simulink model "simVSG"  (R2023a)
settings: Solver=VariableStepAuto  StartTime=0.0  StopTime=Tend  MaxStep=Ts/3  RelTol=1e-3
values from neighbouring files (symbols this model uses):
  Cf = 1.3157e-4    (= 0.00013157)    [VSG.m]
  Dp0 = 3    [VSG.m]
  Fg = 50    [VSG.m]
  Fsw = 2.5e3    (= 2500)    [VSG.m]
  J0 = 3.0/Jn    (= 1.23370055014)    [VSG.m]
  Kd = 150    [VSG.m]
  Kii = Rf*alpha_i / Zn    (= 0.654498469498)    [VSG.m]
  Kj = 30    [VSG.m]
  Kpi = Lf*alpha_i / Zn    (= 0.208332452222)    [VSG.m]
  Kpv = alpha_v*sqrt(alpha_v^2+alpha_i^2)/alpha_i *Zn    [VSG.m]
  Lf = 5.7773e-4    (= 0.00057773)    [VSG.m]
  Pn = 120    [VSG.m]
  Rf = 1.815e-3    (= 0.001815)    [VSG.m]
  Ts = 5e-05    [VSG.m]
  Udc = 800    [VSG.m]
  Ug = 220    [VSG.m]
  Z1 = .09 + 1j*.12    [VSG.m]
  Z3 = .1 + 1j*1.5    [VSG.m]
  Zn = 3*Ug^2 / Pn/1e3    (= 1.21)    [VSG.m]
undefined symbols (not defined in the file or in its folder): DiscIntNeverNeededParam, Vnom_prim
libraries: spsSecondOrderFilterLib x8, simulink x8, spsFirstOrderFilterLib x6, spsThreePhaseSeriesRLCBranchLib x4, spsThreePhaseSeriesRLCLoadLib x3, slpidlib x3, spsThreePhaseVIMeasurementLib x3, spsGroundLib x2, spsPowerPLLDrivenPositiveSequenceLib x2, spsabctodq0Lib x2, spsFundamentalPLLDrivenLib x2, spsPLL3phLib x2
(part 1 of 2)
settings Model: Creator=si  LastModifiedBy=si

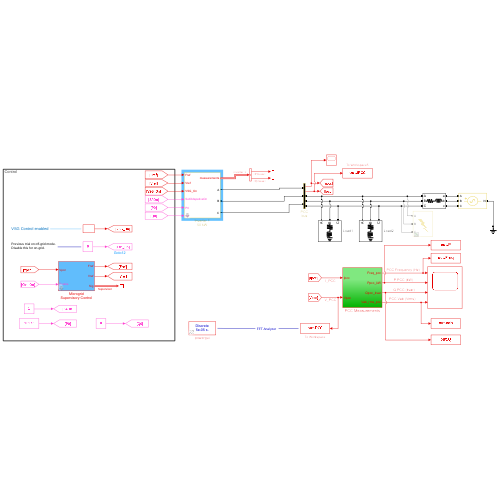
[thumbnail: Simulink's stored preview of the top-level diagram]
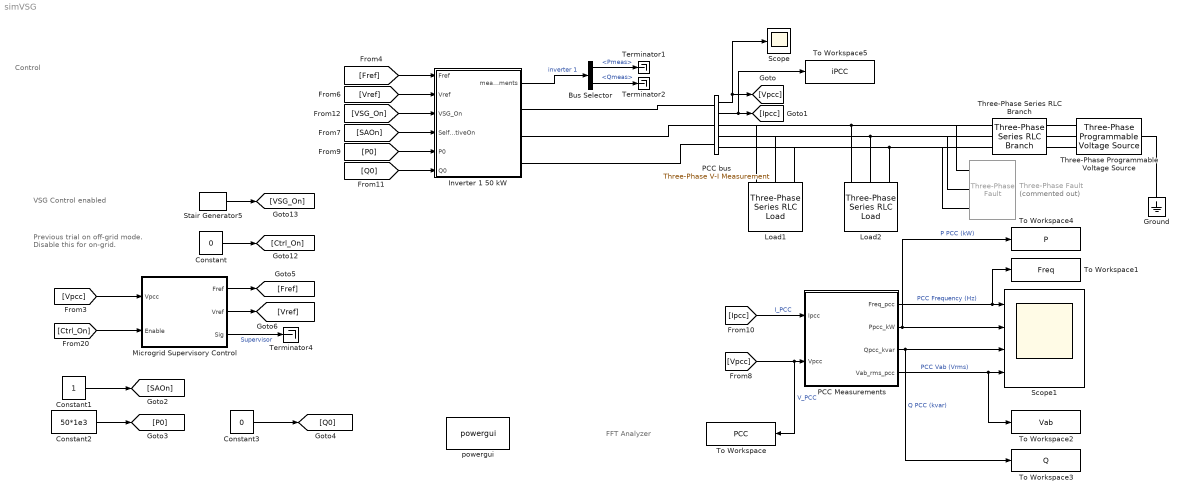
== system simVSG ==
  note: Previous trial on off-grid mode. Disable this for on-grid.
  note: VSG Control enabled
  note: Control
  note: FFT Analyzer
  Bus Selector : BusSelector  OutputSignals=Control.Pmeas,Control.Qmeas
  Constant : Constant  Value=0
  Constant1 : Constant
  Constant2 : Constant  Value=50*1e3
  Constant3 : Constant  Value=0
  Ground : spsGroundLib/Ground  LConnTagsString=a
  Inverter 1 50 kW : Subsystem  mask(Grid-Forming Inverter with droop control){Pnom=Pn*1e3, Fnom=Fg, Vnom=Ug*sqrt(3), Vnom_dc=Udc, Frequency_Droop=25, Voltage_Droop=10, Kp_Vreg=Kpv, Ki_Vreg=0, Kp_Ireg=Kpi, Ki_Ireg=Kii, RLff=[ Rf/Zn, Lf/Zn*2*pi], Fsw=Fsw, CarrierPhase=90, fn_Filter=400, Ts=Ts, ZL=Z1, J0=J0, Dp0=Dp0, Kj=Kj, Kd=Kd, Lv=imag(Z1) / (2*pi*Fg), Rv=real(Z1)}
      mask prompts: Pnom "Power (VA)"; Fnom "Frequency (Hz)"; Vnom "Primary line voltage (Vrms)"; Vnom_dc "DC link voltage (V)"; Frequency_Droop "Frequency droop (%)"; Voltage_Droop "Voltage droop (%)"; Kp_Vreg "Proportional gain"; Ki_Vreg "Integral gain"; Kp_Ireg "Proportional gain"; Ki_Ireg "Integral gain"; RLff "Feedforward coefficients (pu)"; Fsw "Switching frequency (Hz)"; CarrierPhase "Carrier initial phase (degrees)"; fn_Filter "Measurement filters fn (Hz)"; Ts "Sample time (s)"; ZL "Line impedance"; J0 "Initial virtual inertia"; Dp0 "Initial damping factor"; Kj "Inertial changing rate Kj"; Kd "Damping factor changing rate Kd"; Lv "Virtual inductance"; Rv "Virtual resistance"
      mask init:
      | Rff=RLff(1);
      | Lff=RLff(2);
      mask DialogControl Container4 Prompt: Nominal Values:
      mask DialogControl Container8 Prompt: Droop Values
      mask DialogControl Container7 Prompt: Voltage Regulators
      mask DialogControl Container10 Prompt: Current Regulators
      mask DialogControl Ts1 Prompt: PWM Generator
      mask DialogControl Container9 Prompt: Line impedance
      mask DialogControl Container11 Prompt: VSG parameters
  Load1 : spsThreePhaseSeriesRLCLoadLib/Three-Phase Series RLC Load  LConnTagsString=A|B|C  Configuration=Y (grounded)  NominalVoltage=Ug*sqrt(3)  Vabc=[1e3 1e3 1e3]  Vabcp=[1e3 1e3 1e3]  NominalFrequency=Fg  UnbalancedPower=off  ActivePower=40e3  InductivePower=10e3  CapacitivePower=0  Pabc=[10e3 9e3 11e3]  QLabc=[100 90 110]  QCabc=[100 90 110]  Pabcp=[10e3 9e3 11e3]  QLabcp=[100 90 110]  QCabcp=[100 90 110]  Measurements=None  LoadType=constant Z
  Load2 : spsThreePhaseSeriesRLCLoadLib/Three-Phase Series RLC Load  LConnTagsString=A|B|C  Configuration=Y (grounded)  NominalVoltage=Ug*sqrt(3)  Vabc=[1e3 1e3 1e3]  Vabcp=[1e3 1e3 1e3]  NominalFrequency=Fg  UnbalancedPower=off  ActivePower=2e3  InductivePower=6e3  CapacitivePower=0  Pabc=[10e3 9e3 11e3]  QLabc=[100 90 110]  QCabc=[100 90 110]  Pabcp=[10e3 9e3 11e3]  QLabcp=[100 90 110]  QCabcp=[100 90 110]  Measurements=None  LoadType=constant Z
  Microgrid Supervisory Control : Subsystem  mask(Microgrid Supervisory Control){Fnom=Fg, Vnom=Ug*sqrt(3), Kp_Freg=0.03, Ki_Freg=2, Freg_Limits=[1.05, 0.95] * Fg, Kp_Vreg=0.1, Ki_Vreg=7, Vreg_Limits=[1.05, 0.95] * Ug*sqrt(3), fn_Filter=10, Ts=Ts}
      mask prompts: Fnom "Frequency (Hz)"; Vnom "Line voltage (Vrms)"; Kp_Freg "Proportional gain"; Ki_Freg "Integral gain"; Freg_Limits "Output limits (Hz): [Upper Lower]"; Kp_Vreg "Proportional gain"; Ki_Vreg "Integral gain"; Vreg_Limits "Output limits (Hz): [Upper Lower]"; fn_Filter "Measurement filter fn (Hz)"; Ts "Sample time (s)"
      mask DialogControl Container4 Prompt: Nominal Values:
      mask DialogControl Container7 Prompt: Frequency Regulator
      mask DialogControl Container10 Prompt: Voltage Regulator
  PCC bus : spsThreePhaseVIMeasurementLib/Three-Phase V-I Measurement  VoltageMeasurement=phase-to-ground  SetLabelV=off  LabelV=Vabc  Vpu=off  VpuLL=off  CurrentMeasurement=yes  SetLabelI=off  LabelI=Iabc  Ipu=off  Pbase=100e6  Vbase=500e3  OutputType=Complex  PhasorSimulation=off  PSBequivalent=0
  PCC Measurements : Subsystem
  Scope : Scope
  Scope1 : Scope  NumInputPorts=4
  Stair Generator5 : spsStairGeneratorLib/Stair Generator  t=[0, Ts]  e=[0, 1]  Ts=Ts
  Terminator1 : Terminator
  Terminator2 : Terminator
  Terminator4 : Terminator
  Three-Phase Programmable Voltage Source : spsThreePhaseProgrammableVoltageSourceLib/Three-Phase Programmable Voltage Source  PositiveSequence="[Ug*sqrt(3)*1.05  0 Fg]"  VariationEntity=Amplitude  VariationType=Table of time-amplitude pairs  VariationTypeAlt=Ramp  VariationStep=0.5  VariationRate=-.5  VariationMagnitude=0.3  VariationFrequency=2  VariationTiming=[5 5.1]  VariationPhaseA=off  Amplitudes=[1 1 0.5]  TimeValues=[0 4 5]  HarmonicGeneration=off  HarmonicA=[3 0.2 -25 0]  HarmonicB=[2 0.15 35 2]  Timing="[0.05  3]"  BusType=swing  Pref=0  Qref=0  Qmin=-inf  Qmax=inf
  Three-Phase Series RLC Branch : spsThreePhaseSeriesRLCBranchLib/Three-Phase Series RLC Branch  LConnTagsString=A|B|C  RConnTagsString=A|B|C  BranchType=RL  Resistance=real(Z3)  Inductance=imag(Z3)/2/pi/Fg  Capacitance=1e-6  Measurements=None
  Three-Phase Fault : spsThreePhaseFaultLib/Three-Phase Fault  Commented=on  InitialStates=0  FaultA=on  FaultB=off  FaultC=off  GroundFault=on  SwitchTimes=[5 10]  External=off  SwitchStatus=NaN  FaultResistance=0.001  GroundResistance=0.01  SnubberResistance=1e6  SnubberCapacitance=inf  Measurements=None
  To Workspace : ToWorkspace  VariableName=PCC  SaveFormat=Structure With Time  SampleTime=-1
  To Workspace1 : ToWorkspace  VariableName=Freq  SaveFormat=Structure With Time  SampleTime=-1
  To Workspace2 : ToWorkspace  VariableName=Vab  SaveFormat=Structure With Time  SampleTime=-1
  To Workspace3 : ToWorkspace  VariableName=Q  SaveFormat=Structure With Time  SampleTime=-1
  To Workspace4 : ToWorkspace  VariableName=P  SaveFormat=Structure With Time  SampleTime=-1
  To Workspace5 : ToWorkspace  VariableName=iPCC  SaveFormat=Structure With Time  SampleTime=-1
  powergui : spspowerguiLib/powergui  Priority=2  SimulationMode=Discrete  SampleTime=Ts  frequency=60  Iterations=50  frequencyindice=0  Pbase=100e6  ErrMax=1e-4  UnitsV=kV  UnitsW=MW  buscounter=4  FunctionMessages=off  echomessages=off  EnableUseOfTLC=off  CurrentSourceSwitches=off  DisableSnubberDevices=off  DisableRonSwitches=off  DisableVfSwitches=off  DisplayEquations=off  AutomaticDiscreteSolvers=off  SolverType=Tustin/Backward Euler (TBE)  Interpol=off  ExternalGateDelay=off  methode=off  Ts=0  x0status=blocks  SPID=off  SwTol=0  HookPort=off  NonlinearTolerance=1e-4  nMaxIteration=100  ContinueOnMaxIteration=on  RestoreLinks=warning  ResistiveCurrentMeasurement=off  Frange=[0:2:500]  Ylog=off  Xlog=off  ShowGrid=off  save=off  variable=ZData  structure=ScopeData_VIpcc  ZoomFFT=on  StartTime=6.8  cycles=1  DisplayStyle=1  fundamental=60  FreqAxis=off  MaxFrequency=7000  frequencyindicesteady=1  RmsSteady=1  display=off
  wires:
  PCC bus/2 -> To Workspace5/1, [Ipcc]
  Microgrid Supervisory Control/2(Vref) -> [Vref]
  [Ipcc] -> PCC Measurements/1(Ipcc)  "I_PCC"
  Inverter 1 50 kW/1(measurements) -> Bus Selector/1  "inverter 1"
  [Vref] -> Inverter 1 50 kW/2(Vref)
  Microgrid Supervisory Control/3(Sig) -> Terminator4/1  "Supervisor"
  PCC Measurements/2(Ppcc_kW) -> To Workspace4/1, Scope1/2  "P PCC (kW)"
  PCC Measurements/4(Vab_rms_pcc) -> To Workspace2/1, Scope1/4  "PCC Vab (Vrms)"
  [VSG_On] -> Inverter 1 50 kW/3(VSG_On)
  Bus Selector/2 -> Terminator2/1  "<Qmeas>"
  [Fref] -> Inverter 1 50 kW/1(Fref)
  Microgrid Supervisory Control/1(Fref) -> [Fref]
  Bus Selector/1 -> Terminator1/1  "<Pmeas>"
  PCC Measurements/3(Qpcc_kvar) -> To Workspace3/1, Scope1/3  "Q PCC (kvar)"
  [Vpcc] -> Microgrid Supervisory Control/1(Vpcc)
  PCC Measurements/1(Freq_pcc) -> To Workspace1/1, Scope1/1  "PCC Frequency (Hz)"
  Stair Generator5/1 -> [VSG_On]
  [Ctrl_On] -> Microgrid Supervisory Control/2(Enable)
  [Vpcc] -> To Workspace/1, PCC Measurements/2(Vpcc)  "V_PCC"
  PCC bus/1 -> Scope/1, [Vpcc]
  Constant/1 -> [Ctrl_On]
  Constant1/1 -> [SAOn]
  [SAOn] -> Inverter 1 50 kW/4(SelfAdapativeOn)
  Constant2/1 -> [P0]
  [P0] -> Inverter 1 50 kW/5(P0)
  Constant3/1 -> [Q0]
  [Q0] -> Inverter 1 50 kW/6(Q0)
  connections:
  PCC bus/RConn2 -- Load1/LConn2 -- Three-Phase Fault/LConn2 -- Three-Phase Series RLC Branch/LConn2 -- Load2/LConn2
  PCC bus/RConn3 -- Load1/LConn3 -- Three-Phase Fault/LConn3 -- Three-Phase Series RLC Branch/LConn3 -- Load2/LConn3
  PCC bus/RConn1 -- Load1/LConn1 -- Three-Phase Fault/LConn1 -- Three-Phase Series RLC Branch/LConn1 -- Load2/LConn1
  Inverter 1 50 kW/RConn3 -- PCC bus/LConn3
  Inverter 1 50 kW/RConn2 -- PCC bus/LConn2
  Inverter 1 50 kW/RConn1 -- PCC bus/LConn1
  Ground/LConn1 -- Three-Phase Programmable Voltage Source/LConn1
  Three-Phase Programmable Voltage Source/RConn1 -- Three-Phase Series RLC Branch/RConn1
  Three-Phase Programmable Voltage Source/RConn2 -- Three-Phase Series RLC Branch/RConn2
  Three-Phase Programmable Voltage Source/RConn3 -- Three-Phase Series RLC Branch/RConn3

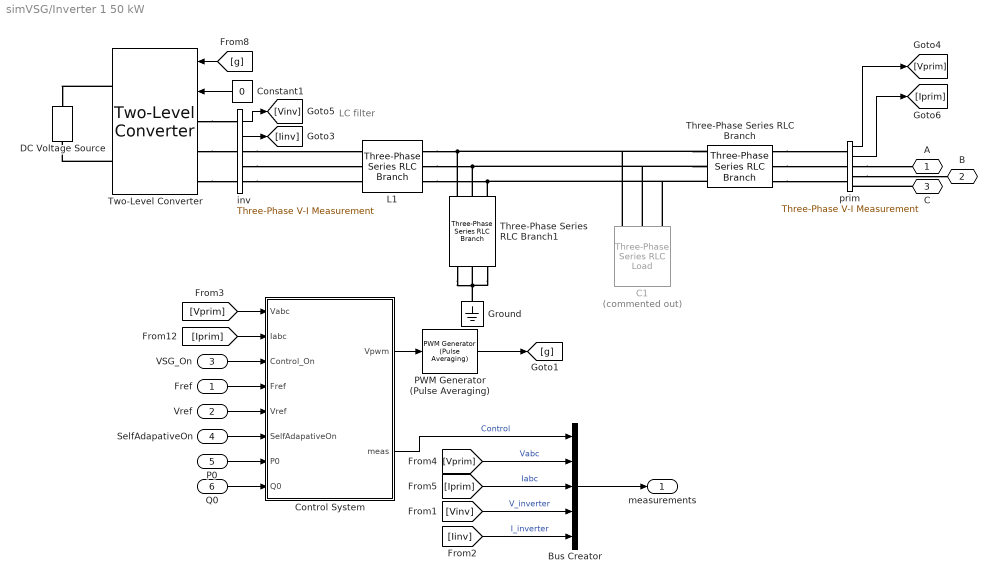
== system simVSG/Inverter 1 50 kW ==
  note: LC filter
  Fref : Inport  PortDimensions=1
  Vref : Inport  Port=2  PortDimensions=1
  VSG_On : Inport  Port=3  PortDimensions=1
  SelfAdapativeOn : Inport  Port=4  PortDimensions=1
  P0 : Inport  Port=5  PortDimensions=1
  Q0 : Inport  Port=6  PortDimensions=1
  Bus Creator : BusCreator  Inputs=5
  C1 : spsThreePhaseSeriesRLCLoadLib/Three-Phase Series RLC Load  Commented=on  LConnTagsString=A|B|C  Configuration=Y (grounded)  NominalVoltage=Vnom  Vabc=[1e3 1e3 1e3]  Vabcp=[1e3 1e3 1e3]  NominalFrequency=Fnom  UnbalancedPower=off  ActivePower=0  InductivePower=0  CapacitivePower=0.05*Pnom  Pabc=[10e3 9e3 11e3]  QLabc=[100 90 110]  QCabc=[100 90 110]  Pabcp=[10e3 9e3 11e3]  QLabcp=[100 90 110]  QCabcp=[100 90 110]  Measurements=None  LoadType=constant Z
  Constant1 : Constant  Value=0
  Control System : Subsystem  mask(Inverter Control){Pnom=Pnom, Fnom=Fnom, Vnom=Vnom, Vnom_dc=Vnom_dc, Frequency_Droop=Frequency_Droop, Voltage_Droop=Voltage_Droop, Kp_Vreg=Kp_Vreg, Ki_Vreg=Ki_Vreg, fn_Filter=fn_Filter, Kp_Ireg=Kp_Ireg, Ki_Ireg=Ki_Ireg, RLff=[ Rff Lff], J0=J0, Dp0=Dp0, Kj=Kj, Kd=Kd, Lv=Lv, Rv=Rv, Ts=Ts}
      mask prompts: Pnom "Power (VA)"; Fnom "Frequency (Hz)"; Vnom "Primary voltage (Vrms)"; Vnom_dc "DC voltage (V)"; Frequency_Droop "Frequency droop (%)"; Voltage_Droop "Voltage droop (%)"; Kp_Vreg "Proportional gain"; Ki_Vreg "Integral gain"; fn_Filter "Measurement filter fn (Hz)"; Kp_Ireg "Proportional gain"; Ki_Ireg "Integral gain"; RLff "Feedforward Values [Rff Lff] (pu)"; J0 "Initial virtual inertia"; Dp0 "Initial damping factor"; Kj "Inertial changing rate Kj"; Kd "Damping factor changing rate Kd"; Lv "Virtual inductance"; Rv "Virtual resistance"; Ts "Control sample time:"
      mask init:
      | Rff=RLff(1);
      | Lff=RLff(2);
      | Limits_Ireg=[1.25, -1.25];
      | Limits_Vreg=[1.25, -1.25];
      mask DialogControl Container4 Prompt: Nominal Values:
      mask DialogControl Container8 Prompt: Droop Values
      mask DialogControl Container9 Prompt: Voltage regulators
      mask DialogControl Container6 Prompt: Current regulators:
      mask DialogControl Container10 Prompt: VSG parameters
      mask DialogControl Ts1 Prompt: Sample time (s)
  DC Voltage Source : spsDCVoltageSourceLib/DC Voltage Source  Amplitude=Vnom_dc  Measurements=None
  Ground : spsGroundLib/Ground  LConnTagsString=a
  L1 : spsThreePhaseSeriesRLCBranchLib/Three-Phase Series RLC Branch  LConnTagsString=A|B|C  RConnTagsString=A|B|C  BranchType=RL  Resistance=Rf  Inductance=Lf  Capacitance=inf  Measurements=None
  PWM Generator (Pulse Averaging) : spsPWMGeneratorPulseAveragingLib/PWM Generator (Pulse Averaging)  GeneratorType=Two-level, three-phase  Fc=Fsw  InitialPhase=CarrierPhase  Ts=Ts
  Three-Phase Series RLC Branch : spsThreePhaseSeriesRLCBranchLib/Three-Phase Series RLC Branch  LConnTagsString=A|B|C  RConnTagsString=A|B|C  BranchType=RL  Resistance=real(ZL)  Inductance=imag(ZL)/2/pi/Fg  Capacitance=1e-6  Measurements=None
  Three-Phase Series RLC Branch1 : spsThreePhaseSeriesRLCBranchLib/Three-Phase Series RLC Branch  LConnTagsString=A|B|C  RConnTagsString=A|B|C  BranchType=C  Resistance=1  Inductance=1e-3  Capacitance=Cf  Measurements=None
  Two-Level Converter : spsTwoLevelConverterLib/Two-Level Converter  ModelType=Switching function  Ron=1e-3  Rs=1e6  Cs=inf  Vforward=[0,0]  Ron_Diode=1e-6  Rs_Diode=1e6  Cs_Diode=1e-06  Vf_Diode=0  Rs_CurrentSource=inf  Ron_ACsource=1e-3
  inv : spsThreePhaseVIMeasurementLib/Three-Phase V-I Measurement  VoltageMeasurement=phase-to-ground  SetLabelV=off  LabelV=Vabc_B1  Vpu=off  VpuLL=off  CurrentMeasurement=yes  SetLabelI=off  LabelI=Iabc_B1  Ipu=off  Pbase=100e6  Vbase=500e3  OutputType=Magnitude  PhasorSimulation=off  PSBequivalent=0
  prim : spsThreePhaseVIMeasurementLib/Three-Phase V-I Measurement  VoltageMeasurement=phase-to-ground  SetLabelV=off  LabelV=Vabc_B1  Vpu=off  VpuLL=off  CurrentMeasurement=yes  SetLabelI=off  LabelI=Iabc_B1  Ipu=off  Pbase=100e6  Vbase=500e3  OutputType=Magnitude  PhasorSimulation=off  PSBequivalent=0
  A : PMIOPort  Side=Right
  B : PMIOPort  Port=2  Side=Right
  C : PMIOPort  Port=3  Side=Right
  measurements : Outport
  wires:
  Bus Creator/1 -> measurements/1
  [Iinv] -> Bus Creator/5  "I_inverter"
  [Vinv] -> Bus Creator/4  "V_inverter"
  [Iprim] -> Bus Creator/3  "Iabc"
  [Vprim] -> Bus Creator/2  "Vabc"
  Control System/1(Vpwm) -> PWM Generator (Pulse Averaging)/1
  inv/2 -> [Iinv]
  PWM Generator (Pulse Averaging)/1 -> [g]
  inv/1 -> [Vinv]
  [g] -> Two-Level Converter/1
  Constant1/1 -> Two-Level Converter/2
  Fref/1 -> Control System/4(Fref)
  Vref/1 -> Control System/5(Vref)
  Control System/2(meas) -> Bus Creator/1  "Control"
  VSG_On/1 -> Control System/3(Control_On)
  prim/2 -> [Iprim]
  prim/1 -> [Vprim]
  [Vprim] -> Control System/1(Vabc)
  [Iprim] -> Control System/2(Iabc)
  SelfAdapativeOn/1 -> Control System/6(SelfAdapativeOn)
  P0/1 -> Control System/7(P0)
  Q0/1 -> Control System/8(Q0)
  connections:
  L1/RConn2 -- Three-Phase Series RLC Branch/LConn2 -- C1/LConn2 -- Three-Phase Series RLC Branch1/LConn2
  L1/RConn1 -- Three-Phase Series RLC Branch/LConn1 -- C1/LConn1 -- Three-Phase Series RLC Branch1/LConn1
  L1/RConn3 -- Three-Phase Series RLC Branch/LConn3 -- C1/LConn3 -- Three-Phase Series RLC Branch1/LConn3
  Two-Level Converter/RConn1 -- DC Voltage Source/RConn1
  inv/RConn3 -- L1/LConn3
  Two-Level Converter/LConn3 -- inv/LConn3
  inv/RConn1 -- L1/LConn1
  Two-Level Converter/LConn2 -- inv/LConn2
  inv/RConn2 -- L1/LConn2
  Two-Level Converter/LConn1 -- inv/LConn1
  prim/RConn1 -- A/RConn1
  prim/RConn2 -- B/RConn1
  C/RConn1 -- prim/RConn3
  Two-Level Converter/RConn2 -- DC Voltage Source/LConn1
  Three-Phase Series RLC Branch/RConn2 -- prim/LConn2
  Three-Phase Series RLC Branch/RConn1 -- prim/LConn1
  Three-Phase Series RLC Branch/RConn3 -- prim/LConn3
  Ground/LConn1 -- Three-Phase Series RLC Branch1/RConn3 -- Three-Phase Series RLC Branch1/RConn1 -- Three-Phase Series RLC Branch1/RConn2

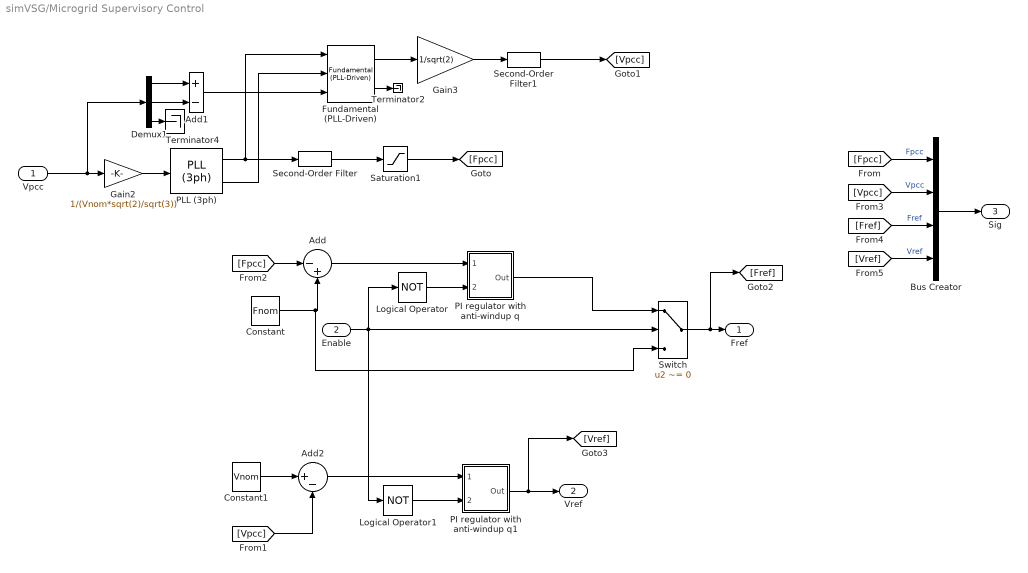
== system simVSG/Microgrid Supervisory Control ==
  Vpcc : Inport
  Enable : Inport  Port=2
  Add : Sum  Inputs=|-+
  Add1 : Sum  Inputs=+-
  Add2 : Sum  Inputs=|+-
  Bus Creator : BusCreator  Inputs=4
  Constant : Constant  Value=Fnom  SampleTime=Ts
  Constant1 : Constant  Value=Vnom  SampleTime=Ts
  Demux1 : Demux  Outputs=3
  Fundamental (PLL-Driven) : spsFundamentalPLLDrivenLib/Fundamental (PLL-Driven)  Finit=Fnom  Fmin=40  InInit=[1, 0]  Ts=Ts
  Gain2 : Gain  Gain=1/(Vnom*sqrt(2)/sqrt(3))
  Gain3 : Gain  Gain=1/sqrt(2)
  Logical Operator : Logic  Operator=NOT  AllPortsSameDT=off  OutDataTypeStr=boolean
  Logical Operator1 : Logic  Operator=NOT  AllPortsSameDT=off  OutDataTypeStr=boolean
  PI regulator with anti-windup q : Subsystem  DialogController=POWERSYS.PowerSysDialog  mask(Discrete PI Controller){Kp=Kp_Freg, Ki=Ki_Freg, Par_Limits=Freg_Limits, Init=Fnom, Ts=Ts}
      mask prompts: Kp "Proportional gain (Kp):"; Ki "Integral gain (Ki):"; Par_Limits "Output limits: [ Upper   Lower ]"; Init "Output initial value:"; Ts "Sample time:"
      mask help: This block implements a discrete PI controller.
      mask init:
      | UpperLimit=Par_Limits(1);
      | LowerLimit=Par_Limits(2);
      | power_initmask();
      mask Help: This block is part of a subset of blocks in the Extras library that does not have documentation associated with it, other than the block mask description.
      mask Display: disp('PI');
  PI regulator with anti-windup q1 : Subsystem  DialogController=POWERSYS.PowerSysDialog  mask(Discrete PI Controller){Kp=Kp_Vreg, Ki=Ki_Vreg, Par_Limits=Vreg_Limits, Init=Vnom, Ts=Ts}
      mask prompts: Kp "Proportional gain (Kp):"; Ki "Integral gain (Ki):"; Par_Limits "Output limits: [ Upper   Lower ]"; Init "Output initial value:"; Ts "Sample time:"
      mask help: This block implements a discrete PI controller.
      mask init:
      | UpperLimit=Par_Limits(1);
      | LowerLimit=Par_Limits(2);
      | power_initmask();
      mask Help: This block is part of a subset of blocks in the Extras library that does not have documentation associated with it, other than the block mask description.
      mask Display: disp('PI');
  PLL (3ph) : spsPLL3phLib/PLL (3ph)  Fmin=40  Par_Init=[0, Fnom]  ParK=[180, 3200, 1]  TcD=1e-4  MaxRateChangeFreq=12  FilterCutOffFreq=20  Ts=Ts  AGC=on
  Saturation1 : Saturate  UpperLimit=1.1*Fnom  LowerLimit=0.9*Fnom
  Second-Order Filter : spsSecondOrderFilterLib/Second-Order Filter  FilterType=Lowpass  Fo=fn_Filter  Zeta=1  Ts=Ts  Initialize=on  Vac_Init="[0,  0,  60]"  Vdc_Init=Fnom  PlotResponse=off  FreqRange=[0, 500, 1]
  Second-Order Filter1 : spsSecondOrderFilterLib/Second-Order Filter  FilterType=Lowpass  Fo=fn_Filter  Zeta=1  Ts=Ts  Initialize=on  Vac_Init="[0,  0,  60]"  Vdc_Init=Vnom  PlotResponse=off  FreqRange=[0, 500, 1]
  Switch : Switch  Criteria=u2 ~= 0  SaturateOnIntegerOverflow=off  InputSameDT=off
  Terminator2 : Terminator
  Terminator4 : Terminator
  Fref : Outport
  Vref : Outport  Port=2
  Sig : Outport  Port=3
  wires:
  [Vpcc] -> Add2/2
  Switch/1 -> [Fref], Fref/1
  Add2/1 -> PI regulator with anti-windup q1/1(Error)
  Second-Order Filter1/1 -> [Vpcc]
  [Fpcc] -> Add/1
  Second-Order Filter/1 -> Saturation1/1
  Saturation1/1 -> [Fpcc]
  Gain3/1 -> Second-Order Filter1/1
  PLL (3ph)/1 -> Fundamental (PLL-Driven)/1, Second-Order Filter/1
  [Vref] -> Bus Creator/4  "Vref"
  [Fpcc] -> Bus Creator/1  "Fpcc"
  [Fref] -> Bus Creator/3  "Fref"
  Demux1/2 -> Add1/2
  Constant/1 -> Switch/3, Add/2
  Demux1/1 -> Add1/1
  PI regulator with anti-windup q/1(Out) -> Switch/1
  Bus Creator/1 -> Sig/1
  PLL (3ph)/2 -> Fundamental (PLL-Driven)/2
  Gain2/1 -> PLL (3ph)/1
  Vpcc/1 -> Gain2/1, Demux1/1
  Fundamental (PLL-Driven)/2 -> Terminator2/1
  [Vpcc] -> Bus Creator/2  "Vpcc"
  Add/1 -> PI regulator with anti-windup q/1(Error)
  Enable/1 -> Logical Operator1/1, Logical Operator/1, Switch/2
  Logical Operator/1 -> PI regulator with anti-windup q/2(Reset)
  Constant1/1 -> Add2/1
  Fundamental (PLL-Driven)/1 -> Gain3/1
  PI regulator with anti-windup q1/1(Out) -> [Vref], Vref/1
  Demux1/3 -> Terminator4/1
  Logical Operator1/1 -> PI regulator with anti-windup q1/2(Reset)
  Add1/1 -> Fundamental (PLL-Driven)/3

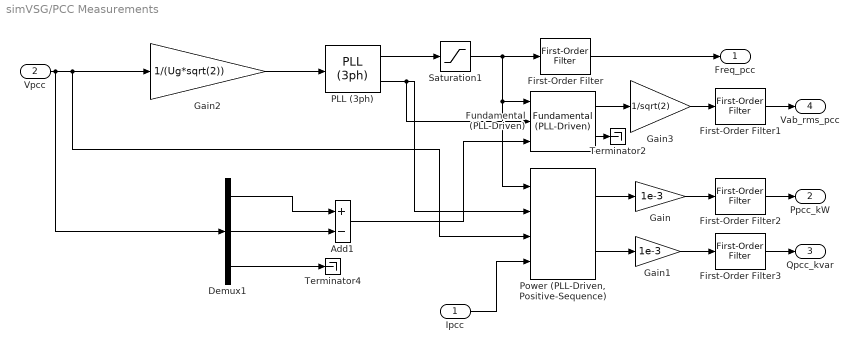
== system simVSG/PCC Measurements ==
  Ipcc : Inport
  Vpcc : Inport  Port=2
  Add1 : Sum  Inputs=+-
  Demux1 : Demux  Outputs=3
  First-Order Filter : spsFirstOrderFilterLib/First-Order Filter  FilterType=Lowpass  Tc=pi/Fg  Ts=Ts  Initialize=on  Vac_Init=[0, 0, Fg]  Vdc_Init=Fg  PlotResponse=off  FreqRange="[0,  200,  1]"
  First-Order Filter1 : spsFirstOrderFilterLib/First-Order Filter  FilterType=Lowpass  Tc=pi/Fg  Ts=Ts  Initialize=on  Vac_Init=[0, 0, Fg]  Vdc_Init=0  PlotResponse=off  FreqRange="[0,  200,  1]"
  First-Order Filter2 : spsFirstOrderFilterLib/First-Order Filter  FilterType=Lowpass  Tc=pi/Fg  Ts=Ts  Initialize=on  Vac_Init=[0, 0, Fg]  Vdc_Init=0  PlotResponse=off  FreqRange="[0,  200,  1]"
  First-Order Filter3 : spsFirstOrderFilterLib/First-Order Filter  FilterType=Lowpass  Tc=pi/Fg  Ts=Ts  Initialize=on  Vac_Init=[0, 0, Fg]  Vdc_Init=0  PlotResponse=off  FreqRange="[0,  200,  1]"
  Fundamental (PLL-Driven) : spsFundamentalPLLDrivenLib/Fundamental (PLL-Driven)  Finit=Fg  Fmin=.8*Fg  InInit=[0, 0]  Ts=Ts
  Gain : Gain  Gain=1e-3
  Gain1 : Gain  Gain=1e-3
  Gain2 : Gain  Gain=1/(Ug*sqrt(2))
  Gain3 : Gain  Gain=1/sqrt(2)
  PLL (3ph) : spsPLL3phLib/PLL (3ph)  Fmin=.8*Fg  Par_Init=[0, Fg]  ParK=[180, 3200, 1]  TcD=1e-4  MaxRateChangeFreq=12  FilterCutOffFreq=20  Ts=Ts  AGC=on
  "Power (PLL-Driven, Positive-Sequence)" : spsPowerPLLDrivenPositiveSequenceLib/Power (PLL-Driven, Positive-Sequence)  Finit=Fg  Fmin=.8*Fg  Vinit=[1, 0]  Iinit=[1, 0]  Ts=Ts
  Saturation1 : Saturate  UpperLimit=1.2*Fg  LowerLimit=.8*Fg
  Terminator2 : Terminator
  Terminator4 : Terminator
  Freq_pcc : Outport
  Ppcc_kW : Outport  Port=2
  Qpcc_kvar : Outport  Port=3
  Vab_rms_pcc : Outport  Port=4
  wires:
  Gain/1 -> First-Order Filter2/1
  "Power (PLL-Driven, Positive-Sequence)"/2 -> Gain1/1
  Gain1/1 -> First-Order Filter3/1
  Gain3/1 -> First-Order Filter1/1
  Vpcc/1 -> Gain2/1, "Power (PLL-Driven, Positive-Sequence)"/3, Demux1/1
  Gain2/1 -> PLL (3ph)/1
  PLL (3ph)/2 -> "Power (PLL-Driven, Positive-Sequence)"/2, Fundamental (PLL-Driven)/2
  Demux1/1 -> Add1/1
  Demux1/3 -> Terminator4/1
  Ipcc/1 -> "Power (PLL-Driven, Positive-Sequence)"/4
  Demux1/2 -> Add1/2
  PLL (3ph)/1 -> Saturation1/1
  Add1/1 -> Fundamental (PLL-Driven)/3
  "Power (PLL-Driven, Positive-Sequence)"/1 -> Gain/1
  Saturation1/1 -> "Power (PLL-Driven, Positive-Sequence)"/1, Fundamental (PLL-Driven)/1, First-Order Filter/1
  Fundamental (PLL-Driven)/2 -> Terminator2/1
  Fundamental (PLL-Driven)/1 -> Gain3/1
  First-Order Filter/1 -> Freq_pcc/1
  First-Order Filter1/1 -> Vab_rms_pcc/1
  First-Order Filter2/1 -> Ppcc_kW/1
  First-Order Filter3/1 -> Qpcc_kvar/1

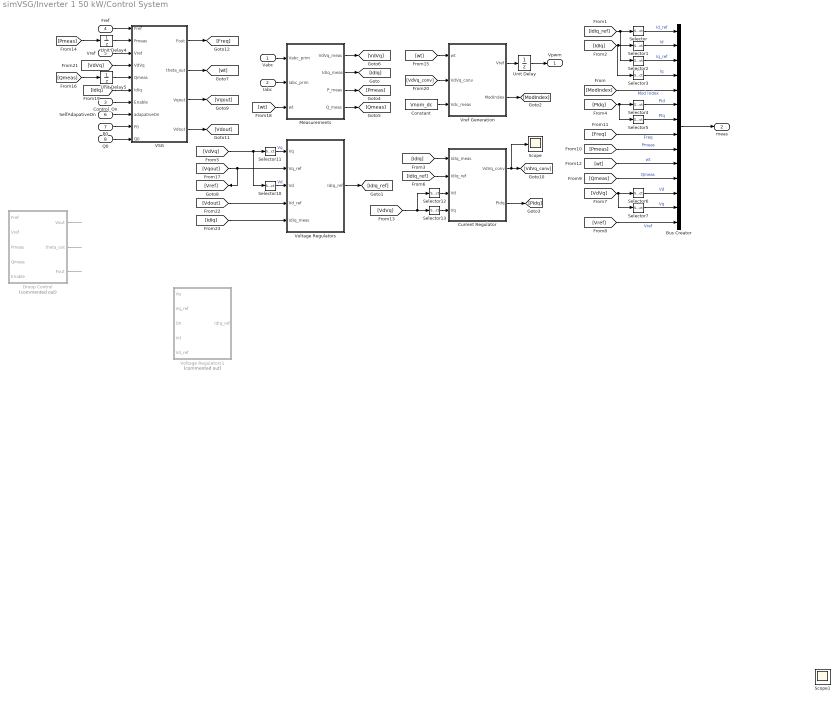
== system simVSG/Inverter 1 50 kW/Control System ==
  Vabc : Inport  PortDimensions=3
  Iabc : Inport  Port=2  PortDimensions=3
  Control_On : Inport  Port=3
  Fref : Inport  Port=4  PortDimensions=1
  Vref : Inport  Port=5  PortDimensions=1
  SelfAdapativeOn : Inport  Port=6
  P0 : Inport  Port=7
  Q0 : Inport  Port=8
  Bus Creator : BusCreator  Inputs=14
  Constant : Constant  Value=Vnom_dc  SampleTime=Ts
  Current Regulator : Subsystem
  Droop Control : Subsystem  Commented=on
  Measurements : Subsystem
  Scope : Scope
  Scope1 : Scope
  Selector{,1,4,6,10,12} (6 alike) : Selector  InputPortWidth=2  IndexOptions=Index vector (dialog)  Indices=1  OutputSizes=1
  Selector{2..3,5,7,11,13} (6 alike) : Selector  InputPortWidth=2  IndexOptions=Index vector (dialog)  Indices=2  OutputSizes=1
  Unit Delay : UnitDelay  SampleTime=-1  HasFrameUpgradeWarning=on
  Unit Delay4 : UnitDelay  SampleTime=-1  HasFrameUpgradeWarning=on
  Unit Delay5 : UnitDelay  SampleTime=-1  HasFrameUpgradeWarning=on
  VSG : Subsystem
  Voltage Regulators : Subsystem
  Voltage Regulators1 : Subsystem  Commented=on
  Vref Generation : Subsystem
  Vpwm : Outport  VectorParamsAs1DForOutWhenUnconnected=off
  meas : Outport  Port=2  VectorParamsAs1DForOutWhenUnconnected=off
  wires:
  Selector1/1 -> Bus Creator/2  "Id"
  Selector5/1 -> Bus Creator/7  "PIq"
  Selector4/1 -> Bus Creator/6  "PId"
  Vref Generation/1(Vref) -> Unit Delay/1
  Vref Generation/2(ModIndex) -> [ModIndex]
  [IdIq] -> Selector1/1, Selector3/1
  [Qmeas] -> Bus Creator/11  "Qmeas"
  Selector/1 -> Bus Creator/1  "Id_ref"
  [Freq] -> Bus Creator/8  "Freq"
  [wt] -> Bus Creator/10  "wt"
  Selector2/1 -> Bus Creator/3  "Iq_ref"
  Measurements/4(Q_meas) -> [Qmeas]
  [IdIq_ref] -> Current Regulator/2(IdIq_ref)
  [PIdq] -> Selector5/1, Selector4/1
  [Pmeas] -> Bus Creator/9  "Pmeas"
  Vabc/1 -> Measurements/1(Vabc_prim)
  Current Regulator/2(PIdq) -> [PIdq]
  [Vqout] -> [Vref], Voltage Regulators/2(Vq_ref)
  [IdIq_ref] -> Selector2/1, Selector/1
  [ModIndex] -> Bus Creator/5  "Mod Index"
  Selector3/1 -> Bus Creator/4  "Iq"
  Constant/1 -> Vref Generation/3(Vdc_meas)
  Bus Creator/1 -> meas/1
  Selector6/1 -> Bus Creator/12  "Vd"
  Selector7/1 -> Bus Creator/13  "Vq"
  [VdVq] -> Selector7/1, Selector6/1
  [Vref] -> Bus Creator/14  "Vref"
  Measurements/1(VdVq_meas) -> [VdVq]
  Measurements/2(IdIq_meas) -> [IdIq]
  [IdIq] -> Current Regulator/1(IdIq_meas)
  Droop Control/3(Fout) -> ?
  Droop Control/1(Vout) -> ?
  Droop Control/2(theta_out) -> ?
  [wt] -> Vref Generation/1(wt)
  [wt] -> Measurements/3(wt)
  Measurements/3(P_meas) -> [Pmeas]
  Unit Delay/1 -> Vpwm/1
  Current Regulator/1(VdVq_conv) -> Scope/1, [VdVq_conv]
  [VdVq_conv] -> Vref Generation/2(VdVq_conv)
  Voltage Regulators/1(IdIq_ref) -> [IdIq_ref]
  Iabc/1 -> Measurements/2(Iabc_prim)
  VSG/1(Fout) -> [Freq]
  VSG/2(theta_out) -> [wt]
  [VdVq] -> VSG/4(VdVq)
  VSG/3(Vqout) -> [Vqout]
  [Qmeas] -> Unit Delay5/1
  [Pmeas] -> Unit Delay4/1
  Vref/1 -> VSG/3(Vref)
  Fref/1 -> VSG/1(Fref)
  Unit Delay5/1 -> VSG/5(Qmeas)
  Unit Delay4/1 -> VSG/2(Pmeas)
  Control_On/1 -> VSG/7(Enable)
  [Vdout] -> Voltage Regulators/4(Vd_ref)
  [IdIq] -> VSG/6(IdIq)
  VSG/4(Vdout) -> [Vdout]
  SelfAdapativeOn/1 -> VSG/8(adapativeOn)
  P0/1 -> VSG/9(P0)
  Q0/1 -> VSG/10(Q0)
  [IdIq] -> Voltage Regulators/5(IdIq_meas)
  Selector11/1 -> Voltage Regulators/1(Vq)  "Vq"
  [VdVq] -> Selector10/1, Selector11/1
  Selector10/1 -> Voltage Regulators/3(Vd)  "Vd"
  [VdVq] -> Selector12/1, Selector13/1
  Selector13/1 -> Current Regulator/4(Vq)
  Selector12/1 -> Current Regulator/3(Vd)

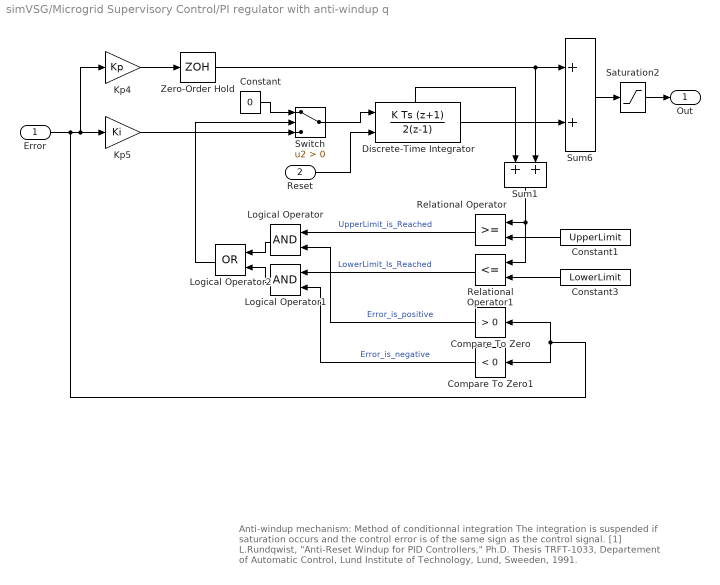
== system simVSG/Microgrid Supervisory Control/PI regulator with anti-windup q ==
  note: Anti-windup mechanism: Method of conditionnal integration
      |
      | The integration is suspended if saturation occurs and the
      | control error is of the same sign as the control signal.
      |
      | [1] L.Rundqwist, "Anti-Reset Windup for PID Controllers," Ph.D. Thesis TRFT-1033,
      | Departement of Automatic Control, Lund Institute of Technology, Lund, Sweeden, 1991.
  Error : Inport  SampleTime=Ts
  Reset : Inport  Port=2  SampleTime=Ts
  Compare To Zero : simulink/Logic and Bit Operations/Compare To Zero  relop=>  OutDataTypeStr=uint8  ZeroCross=off
  Compare To Zero1 : simulink/Logic and Bit Operations/Compare To Zero  relop=<  OutDataTypeStr=uint8  ZeroCross=off
  Constant : Constant  Value=0
  Constant1 : Constant  Value=UpperLimit
  Constant3 : Constant  Value=LowerLimit
  Discrete-Time Integrator : DiscreteIntegrator  IntegratorMethod=Integration: Trapezoidal  ExternalReset=level  InitialCondition=Init  SampleTime=Ts  LimitOutput=on  UpperSaturationLimit=UpperLimit  LowerSaturationLimit=LowerLimit  ShowStatePort=on  ICPrevOutput=DiscIntNeverNeededParam  ICPrevScaledInput=DiscIntNeverNeededParam
  Kp4 : Gain  Gain=Kp  SaturateOnIntegerOverflow=on  SampleTime=Ts  OutDataTypeStr=Inherit: Same as input  ParamDataTypeStr=Inherit: Same as input
  Kp5 : Gain  Gain=Ki  SaturateOnIntegerOverflow=on  SampleTime=Ts  OutDataTypeStr=Inherit: Same as input  ParamDataTypeStr=Inherit: Same as input
  Logical Operator : Logic  AllPortsSameDT=off  OutDataTypeStr=boolean
  Logical Operator1 : Logic  AllPortsSameDT=off  OutDataTypeStr=boolean
  Logical Operator2 : Logic  Operator=OR  AllPortsSameDT=off  OutDataTypeStr=boolean
  Relational Operator : RelationalOperator  OutDataTypeStr=boolean  InputSameDT=off
  Relational Operator1 : RelationalOperator  Operator=<=  OutDataTypeStr=boolean  InputSameDT=off
  Saturation2 : Saturate  UpperLimit=UpperLimit  LowerLimit=LowerLimit
  Sum1 : Sum  InputSameDT=on  SaturateOnIntegerOverflow=on  SampleTime=Ts  OutDataTypeStr=Inherit: Same as first input
  Sum6 : Sum  InputSameDT=on  SaturateOnIntegerOverflow=on  SampleTime=Ts  OutDataTypeStr=Inherit: Same as first input
  Switch : Switch  Criteria=u2 > Threshold  SaturateOnIntegerOverflow=off  InputSameDT=off
  Zero-Order Hold : ZeroOrderHold  SampleTime=Ts
  Out : Outport  SampleTime=Ts  InitialOutput=0  VectorParamsAs1DForOutWhenUnconnected=off
  wires:
  Reset/1 -> Discrete-Time Integrator/2
  Constant/1 -> Switch/1
  Zero-Order Hold/1 -> Sum1/2, Sum6/1
  Discrete-Time Integrator/State -> Sum1/1
  Sum1/1 -> Relational Operator1/1, Relational Operator/1
  Logical Operator2/1 -> Switch/2
  Relational Operator/1 -> Logical Operator/1  "UpperLimit_is_Reached"
  Relational Operator1/1 -> Logical Operator1/1  "LowerLimit_Is_Reached"
  Constant1/1 -> Relational Operator/2
  Constant3/1 -> Relational Operator1/2
  Compare To Zero/1 -> Logical Operator/2  "Error_is_positive"
  Logical Operator/1 -> Logical Operator2/1
  Logical Operator1/1 -> Logical Operator2/2
  Compare To Zero1/1 -> Logical Operator1/2  "Error_is_negative"
  Error/1 -> Compare To Zero1/1, Compare To Zero/1, Kp4/1, Kp5/1
  Sum6/1 -> Saturation2/1
  Kp4/1 -> Zero-Order Hold/1
  Discrete-Time Integrator/1 -> Sum6/2
  Saturation2/1 -> Out/1
  Switch/1 -> Discrete-Time Integrator/1
  Kp5/1 -> Switch/3

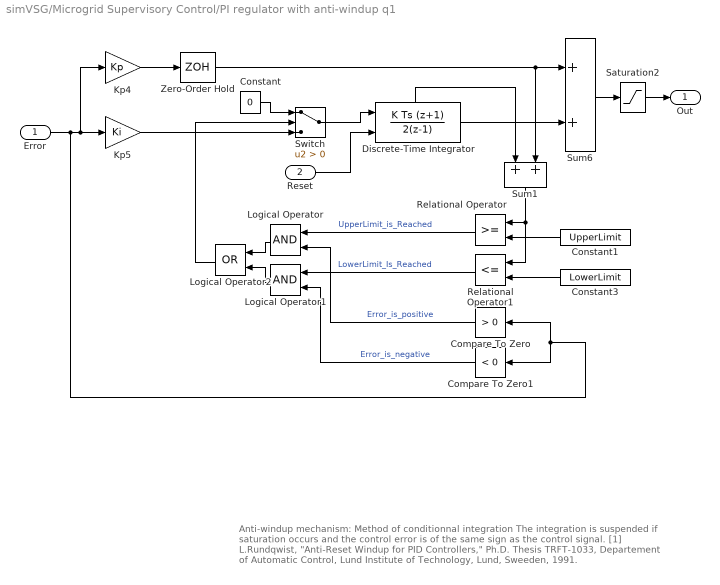
== system simVSG/Microgrid Supervisory Control/PI regulator with anti-windup q1 ==
  note: Anti-windup mechanism: Method of conditionnal integration
      |
      | The integration is suspended if saturation occurs and the
      | control error is of the same sign as the control signal.
      |
      | [1] L.Rundqwist, "Anti-Reset Windup for PID Controllers," Ph.D. Thesis TRFT-1033,
      | Departement of Automatic Control, Lund Institute of Technology, Lund, Sweeden, 1991.
  Error : Inport  SampleTime=Ts
  Reset : Inport  Port=2  SampleTime=Ts
  Compare To Zero : simulink/Logic and Bit Operations/Compare To Zero  relop=>  OutDataTypeStr=uint8  ZeroCross=off
  Compare To Zero1 : simulink/Logic and Bit Operations/Compare To Zero  relop=<  OutDataTypeStr=uint8  ZeroCross=off
  Constant : Constant  Value=0
  Constant1 : Constant  Value=UpperLimit
  Constant3 : Constant  Value=LowerLimit
  Discrete-Time Integrator : DiscreteIntegrator  IntegratorMethod=Integration: Trapezoidal  ExternalReset=level  InitialCondition=Init  SampleTime=Ts  LimitOutput=on  UpperSaturationLimit=UpperLimit  LowerSaturationLimit=LowerLimit  ShowStatePort=on  ICPrevOutput=DiscIntNeverNeededParam  ICPrevScaledInput=DiscIntNeverNeededParam
  Kp4 : Gain  Gain=Kp  SaturateOnIntegerOverflow=on  SampleTime=Ts  OutDataTypeStr=Inherit: Same as input  ParamDataTypeStr=Inherit: Same as input
  Kp5 : Gain  Gain=Ki  SaturateOnIntegerOverflow=on  SampleTime=Ts  OutDataTypeStr=Inherit: Same as input  ParamDataTypeStr=Inherit: Same as input
  Logical Operator : Logic  AllPortsSameDT=off  OutDataTypeStr=boolean
  Logical Operator1 : Logic  AllPortsSameDT=off  OutDataTypeStr=boolean
  Logical Operator2 : Logic  Operator=OR  AllPortsSameDT=off  OutDataTypeStr=boolean
  Relational Operator : RelationalOperator  OutDataTypeStr=boolean  InputSameDT=off
  Relational Operator1 : RelationalOperator  Operator=<=  OutDataTypeStr=boolean  InputSameDT=off
  Saturation2 : Saturate  UpperLimit=UpperLimit  LowerLimit=LowerLimit
  Sum1 : Sum  InputSameDT=on  SaturateOnIntegerOverflow=on  SampleTime=Ts  OutDataTypeStr=Inherit: Same as first input
  Sum6 : Sum  InputSameDT=on  SaturateOnIntegerOverflow=on  SampleTime=Ts  OutDataTypeStr=Inherit: Same as first input
  Switch : Switch  Criteria=u2 > Threshold  SaturateOnIntegerOverflow=off  InputSameDT=off
  Zero-Order Hold : ZeroOrderHold  SampleTime=Ts
  Out : Outport  SampleTime=Ts  InitialOutput=0  VectorParamsAs1DForOutWhenUnconnected=off
  wires:
  Kp5/1 -> Switch/3
  Switch/1 -> Discrete-Time Integrator/1
  Saturation2/1 -> Out/1
  Discrete-Time Integrator/1 -> Sum6/2
  Kp4/1 -> Zero-Order Hold/1
  Sum6/1 -> Saturation2/1
  Error/1 -> Kp5/1, Kp4/1, Compare To Zero/1, Compare To Zero1/1
  Compare To Zero1/1 -> Logical Operator1/2  "Error_is_negative"
  Logical Operator1/1 -> Logical Operator2/2
  Logical Operator/1 -> Logical Operator2/1
  Compare To Zero/1 -> Logical Operator/2  "Error_is_positive"
  Constant3/1 -> Relational Operator1/2
  Constant1/1 -> Relational Operator/2
  Relational Operator1/1 -> Logical Operator1/1  "LowerLimit_Is_Reached"
  Relational Operator/1 -> Logical Operator/1  "UpperLimit_is_Reached"
  Logical Operator2/1 -> Switch/2
  Sum1/1 -> Relational Operator/1, Relational Operator1/1
  Discrete-Time Integrator/State -> Sum1/1
  Zero-Order Hold/1 -> Sum6/1, Sum1/2
  Constant/1 -> Switch/1
  Reset/1 -> Discrete-Time Integrator/2

== system simVSG/Inverter 1 50 kW/Control System/Current Regulator ==
  note: For Ltot >> Rtot :
  note: (Vq_prim - Vq_conv) ~ = - Id * Ltot
  note: (Vd_prim - Vd_conv) ~= + Iq * Ltot
  note: Ltot = Lxfo + Lchoke
      | Rtot = Rxfo + Rchoke
  note: Id positive --> The converter generates active power ("Inverter mode") = Active Power P positive
  note: Iq positive --> The converter absorbs reactive power ("Inductive mode") = Reactive Power Q negative
  note: Sign Convention: Current going out of the converter = positive current
  note: Current Regulator
      | (with feedforward)
  note: Vq_meas + Id*L + Iq*R + deriv(Iq)*L/wbase= Vq_conv
  note: Vd_meas + Id*R - Iq*L + deriv(Id)*L/wbase= Vd_conv
  note: harmonic filter neglected
  IdIq_meas : Inport  PortDimensions=2
  IdIq_ref : Inport  Port=2  PortDimensions=2
  Vd : Inport  Port=3
  Vq : Inport  Port=4
  Add1 : Sum  Inputs=++-
  Add2 : Sum
  Add3 : Sum  Inputs=+++
  Demux1 : Demux  Outputs=2
  Ltot_pu1 : Gain  Gain=Lff*2*pi  SaturateOnIntegerOverflow=on  OutDataTypeStr=Inherit: Same as input  ParamDataTypeStr=Inherit: Same as input
  Ltot_pu2 : Gain  Gain=Lff*2*pi  SaturateOnIntegerOverflow=on  OutDataTypeStr=Inherit: Same as input  ParamDataTypeStr=Inherit: Same as input
  Mux : Mux  Inputs=2
  PID Controller : slpidlib/PID Controller  Controller=PI  Form=Parallel  TimeDomain=Discrete-time  UseExternalTs=off  SampleTime=Ts  IntegratorMethod=Forward Euler  FilterMethod=Forward Euler  ControllerParametersSource=internal  P=Kp_Ireg  I=Ki_Ireg  UseKiTs=off  D=0  N=100  UseFilter=on  TunerSelectOption=Transfer Function Based (PID Tuner App)  InitialConditionSource=internal  InitialConditionForIntegrator=0  InitialConditionForFilter=0  DifferentiatorICPrevScaledInput=0  ExternalReset=none  TrackingMode=off  Kt=1  LimitOutput=on  SatLimitsSource=internal  UpperSaturationLimit=Limits_Ireg(1)  LowerSaturationLimit=Limits_Ireg(2)  LinearizeAsGain=on  AntiWindupMode=clamping  Kb=1  LimitIntegrator=off  UpperIntegratorSaturationLimit=inf  LowerIntegratorSaturationLimit=-inf  POutMin=[]  POutMax=[]  IOutMin=[]  IOutMax=[]  DOutMin=[]  DOutMax=[]  NOutMin=[]  NOutMax=[]  SumOutMin=[]  SumOutMax=[]  SaturationOutMin=[]  SaturationOutMax=[]  PParamMin=[]  PParamMax=[]  IParamMin=[]  IParamMax=[]  DParamMin=[]  DParamMax=[]  NParamMin=[]  NParamMax=[]  KbParamMin=[]  KbParamMax=[]  KtParamMin=[]  KtParamMax=[]  KbOutMin=[]  KbOutMax=[]  KtOutMin=[]  KtOutMax=[]  IntegratorOutMin=[]  IntegratorOutMax=[]  FilterOutMin=[]  FilterOutMax=[]  SumI1OutMin=[]  SumI1OutMax=[]  SumI2OutMin=[]  SumI2OutMax=[]  SumI3OutMin=[]  SumI3OutMax=[]  SumI4OutMin=[]  SumI4OutMax=[]  SumDOutMin=[]  SumDOutMax=[]  DifferentiatorOutMin=[]  DifferentiatorOutMax=[]  FilterDiffOutCoefMin=[]  FilterDiffOutCoefMax=[]  ReciprocalOutMin=[]  ReciprocalOutMax=[]  SumDenOutMin=[]  SumDenOutMax=[]  SumNumOutMin=[]  SumNumOutMax=[]  DivideOutMin=[]  DivideOutMax=[]  UdiffTsProdOutMin=[]  UdiffTsProdOutMax=[]  NTsProdOutMin=[]  NTsProdOutMax=[]  UintegralTsProdOutMin=[]  UintegralTsProdOutMax=[]  UngainTsProdOutMin=[]  UngainTsProdOutMax=[]  ClampingZeroOutDataTypeStr=Inherit: Inherit via back propagation  ClampingZeroOutMin=[]  ClampingZeroOutMax=[]  FilterDenConstantOutDataTypeStr=Inherit: Inherit via back propagation  FilterDenConstantOutMin=[]  FilterDenConstantOutMax=[]  PCopyOutDataTypeStr=Inherit: Inherit via back propagation  PCopyOutMin=[]  PCopyOutMax=[]  NCopyOutDataTypeStr=Inherit: Inherit via back propagation  NCopyOutMin=[]  NCopyOutMax=[]  IntegratorContinuousStateAttributes=''  IntegratorStateMustResolveToSignalObject=off  IntegratorRTWStateStorageClass=Auto  FilterContinuousStateAttributes=''  FilterStateMustResolveToSignalObject=off  FilterRTWStateStorageClass=Auto  ParallelPVariant=InternalParameters  IdealPVariant=Disabled  IVariant=InternalParameters  DVariant=Disabled  IntegratorVariant=Discrete  SatVariant=Enabled  AWVariant=DiscClampingParallel  PCopyVariant=Disabled  TRVariant=Disabled  FdbkBlocksVariant=Forward  IdealPFdbkVariant=Disabled  SatFdbkVariant=Disabled  DerivativeFilterVariant=Disabled  NVariant=Disabled  NCopyVariant=Disabled_SignalSpec  FilterICVariant=Disabled  IntegratorICVariant=InternalICs  ExternalResetVariant=Disabled  TRSumVariant=Passthrough  SumFdbkVariant=Disabled  SumVariant=Sum_PI  TsampFilterVariant=InternalTs  TsampNgainVariant=Passthrough  TsampIntegralVariant=Disabled_SignalSpec  ExternalSaturationOutDataTypeStr=Inherit: Same as second input
  Rtot_pu1 : Gain  Gain=Rff  SaturateOnIntegerOverflow=on  OutDataTypeStr=Inherit: Same as input  ParamDataTypeStr=Inherit: Same as input
  Rtot_pu5 : Gain  Gain=Rff  SaturateOnIntegerOverflow=on  OutDataTypeStr=Inherit: Same as input  ParamDataTypeStr=Inherit: Same as input
  Saturation : Saturate  UpperLimit=Limits_Ireg(1)  LowerLimit=Limits_Ireg(2)
  Sum : Sum  Inputs=|-+
  VdVq_conv : Outport  VectorParamsAs1DForOutWhenUnconnected=off
  PIdq : Outport  Port=2  VectorParamsAs1DForOutWhenUnconnected=off
  wires:
  Add3/1 -> Mux/2
  Vq/1 -> Add3/1
  Add1/1 -> Mux/1  "Feedforward"
  Ltot_pu2/1 -> Add3/3
  Rtot_pu5/1 -> Add3/2
  Demux1/2 -> Rtot_pu5/1, Ltot_pu1/1
  Ltot_pu1/1 -> Add1/3
  Demux1/1 -> Ltot_pu2/1, Rtot_pu1/1
  Rtot_pu1/1 -> Add1/2
  Vd/1 -> Add1/1
  Saturation/1 -> VdVq_conv/1
  Add2/1 -> Saturation/1
  IdIq_meas/1 -> Sum/1
  IdIq_ref/1 -> Demux1/1, Sum/2
  Sum/1 -> PID Controller/1
  PID Controller/1 -> Add2/1, PIdq/1  "PI"
  Mux/1 -> Add2/2

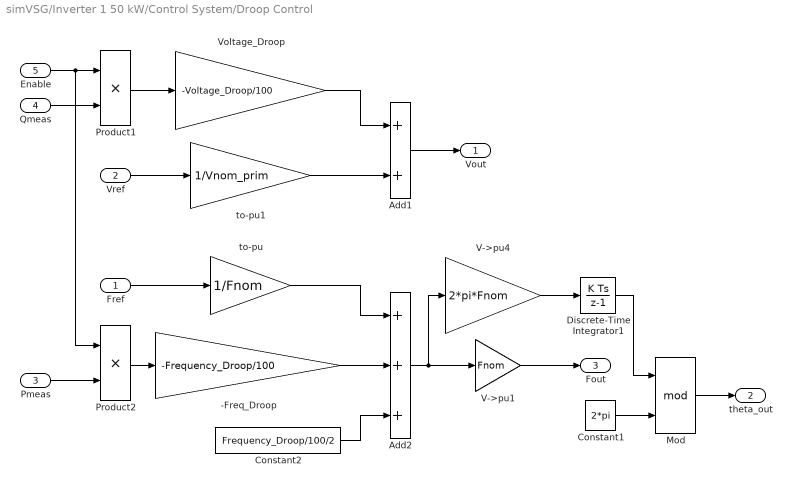
== system simVSG/Inverter 1 50 kW/Control System/Droop Control ==
  Fref : Inport  PortDimensions=1
  Vref : Inport  Port=2  PortDimensions=1
  Pmeas : Inport  Port=3
  Qmeas : Inport  Port=4
  Enable : Inport  Port=5
  -Freq_Droop : Gain  Gain=-Frequency_Droop/100
  Add1 : Sum
  Add2 : Sum  Inputs=+++
  Constant1 : Constant  Value=2*pi
  Constant2 : Constant  Value=Frequency_Droop/100/2
  Discrete-Time Integrator1 : DiscreteIntegrator  SampleTime=Ts  ICPrevOutput=DiscIntNeverNeededParam  ICPrevScaledInput=DiscIntNeverNeededParam
  Mod : Math  Operator=mod
  Product1 : Product
  Product2 : Product
  V->pu1 : Gain  Gain=Fnom  SaturateOnIntegerOverflow=on  OutDataTypeStr=Inherit: Same as input  ParamDataTypeStr=Inherit: Same as input
  V->pu4 : Gain  Gain=2*pi*Fnom  SaturateOnIntegerOverflow=on  OutDataTypeStr=Inherit: Same as input  ParamDataTypeStr=Inherit: Same as input
  Voltage_Droop : Gain  Gain=-Voltage_Droop/100
  to-pu : Gain  Gain=1/Fnom
  to-pu1 : Gain  Gain=1/Vnom_prim
  Vout : Outport
  theta_out : Outport  Port=2
  Fout : Outport  Port=3
  wires:
  Mod/1 -> theta_out/1
  Constant1/1 -> Mod/2
  Discrete-Time Integrator1/1 -> Mod/1
  V->pu1/1 -> Fout/1
  Add2/1 -> V->pu1/1, V->pu4/1
  Enable/1 -> Product2/1, Product1/1
  Pmeas/1 -> Product2/2
  Constant2/1 -> Add2/3
  Fref/1 -> to-pu/1
  Product2/1 -> -Freq_Droop/1
  Vref/1 -> to-pu1/1
  Qmeas/1 -> Product1/2
  -Freq_Droop/1 -> Add2/2
  to-pu1/1 -> Add1/2
  Product1/1 -> Voltage_Droop/1
  Voltage_Droop/1 -> Add1/1
  to-pu/1 -> Add2/1
  V->pu4/1 -> Discrete-Time Integrator1/1
  Add1/1 -> Vout/1

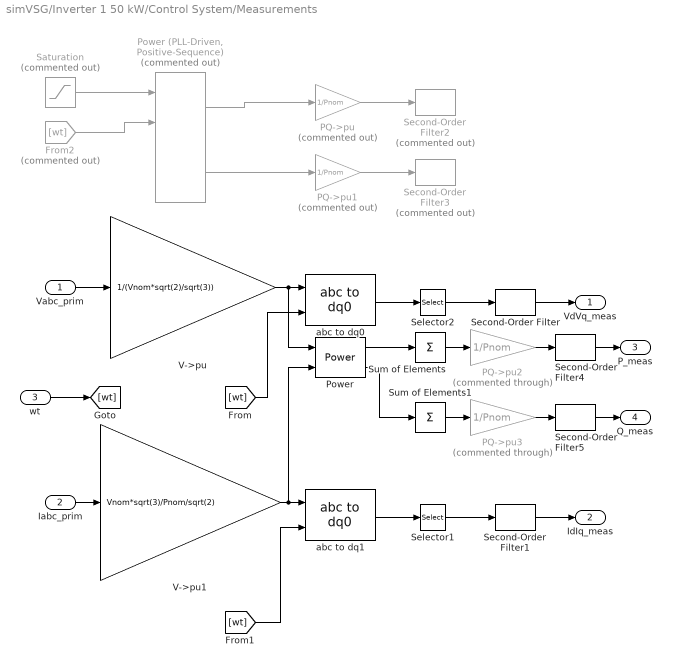
== system simVSG/Inverter 1 50 kW/Control System/Measurements ==
  Vabc_prim : Inport
  Iabc_prim : Inport  Port=2
  wt : Inport  Port=3
  From2 : From  Commented=on  GotoTag=wt
  PQ->pu : Gain  Commented=on  Gain=1/Pnom  SaturateOnIntegerOverflow=on  OutDataTypeStr=Inherit: Same as input  ParamDataTypeStr=Inherit: Same as input
  PQ->pu1 : Gain  Commented=on  Gain=1/Pnom  SaturateOnIntegerOverflow=on  OutDataTypeStr=Inherit: Same as input  ParamDataTypeStr=Inherit: Same as input
  PQ->pu2 : Gain  Commented=through  Gain=1/Pnom  SaturateOnIntegerOverflow=on  OutDataTypeStr=Inherit: Same as input  ParamDataTypeStr=Inherit: Same as input
  PQ->pu3 : Gain  Commented=through  Gain=1/Pnom  SaturateOnIntegerOverflow=on  OutDataTypeStr=Inherit: Same as input  ParamDataTypeStr=Inherit: Same as input
  Power : spsPowerLib/Power  Freq=Fnom  Vinit=[1, 0]  Iinit=[1, 0]  Ts=0
  "Power (PLL-Driven, Positive-Sequence)" : spsPowerPLLDrivenPositiveSequenceLib/Power (PLL-Driven, Positive-Sequence)  Commented=on  Finit=60  Fmin=45  Vinit=[1, 0]  Iinit=[1, 0]  Ts=Ts
  Saturation : Saturate  Commented=on  UpperLimit=65  LowerLimit=55
  Second-Order Filter{,1,4..5} (4 alike) : spsSecondOrderFilterLib/Second-Order Filter  FilterType=Lowpass  Fo=fn_Filter  Zeta=1  Ts=Ts  Initialize=off  Vac_Init="[0,  0,  60]"  Vdc_Init=0  PlotResponse=off  FreqRange=[0, 500, 1]
  Second-Order Filter2 : spsSecondOrderFilterLib/Second-Order Filter  Commented=on  FilterType=Lowpass  Fo=fn_Filter  Zeta=1  Ts=Ts  Initialize=off  Vac_Init="[0,  0,  60]"  Vdc_Init=0  PlotResponse=off  FreqRange=[0, 500, 1]
  Second-Order Filter3 : spsSecondOrderFilterLib/Second-Order Filter  Commented=on  FilterType=Lowpass  Fo=fn_Filter  Zeta=1  Ts=Ts  Initialize=off  Vac_Init="[0,  0,  60]"  Vdc_Init=0  PlotResponse=off  FreqRange=[0, 500, 1]
  Selector1 : Selector  InputPortWidth=3  IndexOptions=Index vector (dialog)  Indices=[1 2]  OutputSizes=1
  Selector2 : Selector  InputPortWidth=3  IndexOptions=Index vector (dialog)  Indices=[1 2]  OutputSizes=1
  Sum of Elements : Sum  Inputs=+
  Sum of Elements1 : Sum  Inputs=+
  V->pu : Gain  Gain=1/(Vnom*sqrt(2)/sqrt(3))  SaturateOnIntegerOverflow=on  OutDataTypeStr=Inherit: Same as input  ParamDataTypeStr=Inherit: Same as input
  V->pu1 : Gain  Gain=Vnom*sqrt(3)/Pnom/sqrt(2)  SaturateOnIntegerOverflow=on  OutDataTypeStr=Inherit: Same as input  ParamDataTypeStr=Inherit: Same as input
  abc to dq0 : spsabctodq0Lib/abc to dq0  Alignment=90 degrees behind phase A axis
  abc to dq1 : spsabctodq0Lib/abc to dq0  Alignment=90 degrees behind phase A axis
  VdVq_meas : Outport  VectorParamsAs1DForOutWhenUnconnected=off
  IdIq_meas : Outport  Port=2  VectorParamsAs1DForOutWhenUnconnected=off
  P_meas : Outport  Port=3  VectorParamsAs1DForOutWhenUnconnected=off
  Q_meas : Outport  Port=4  VectorParamsAs1DForOutWhenUnconnected=off
  wires:
  PQ->pu3/1 -> Second-Order Filter5/1
  PQ->pu2/1 -> Second-Order Filter4/1
  Second-Order Filter/1 -> VdVq_meas/1
  Sum of Elements/1 -> PQ->pu2/1
  Selector2/1 -> Second-Order Filter/1
  abc to dq1/1 -> Selector1/1
  Power/2 -> Sum of Elements1/1
  Selector1/1 -> Second-Order Filter1/1
  abc to dq0/1 -> Selector2/1
  PQ->pu/1 -> Second-Order Filter2/1
  Iabc_prim/1 -> V->pu1/1
  From2/1 -> "Power (PLL-Driven, Positive-Sequence)"/2
  Vabc_prim/1 -> V->pu/1
  V->pu1/1 -> Power/2, abc to dq1/1
  Sum of Elements1/1 -> PQ->pu3/1
  wt/1 -> [wt]
  [wt] -> abc to dq1/2
  "Power (PLL-Driven, Positive-Sequence)"/1 -> PQ->pu/1
  PQ->pu1/1 -> Second-Order Filter3/1
  "Power (PLL-Driven, Positive-Sequence)"/2 -> PQ->pu1/1
  Second-Order Filter1/1 -> IdIq_meas/1
  Power/1 -> Sum of Elements/1
  Saturation/1 -> "Power (PLL-Driven, Positive-Sequence)"/1
  V->pu/1 -> Power/1, abc to dq0/1
  [wt] -> abc to dq0/2
  Second-Order Filter4/1 -> P_meas/1
  Second-Order Filter5/1 -> Q_meas/1

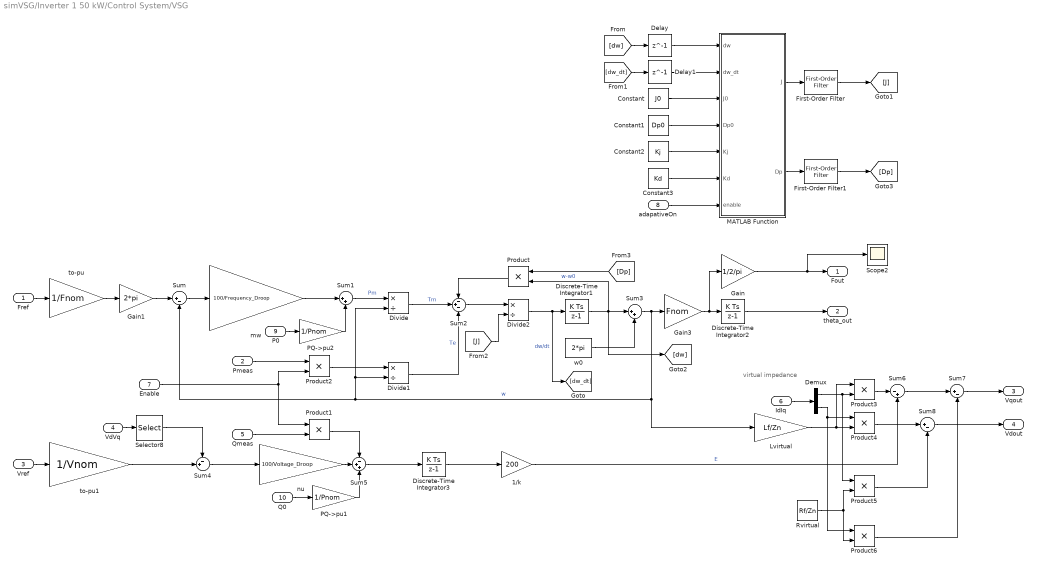
== system simVSG/Inverter 1 50 kW/Control System/VSG ==
  note: virtual impedance
  Fref : Inport
  Pmeas : Inport  Port=2
  Vref : Inport  Port=3
  VdVq : Inport  Port=4
  Qmeas : Inport  Port=5
  IdIq : Inport  Port=6
  Enable : Inport  Port=7
  adapativeOn : Inport  Port=8
  P0 : Inport  Port=9
  Q0 : Inport  Port=10
  1/k : Gain  Gain=200
  Constant : Constant  Value=J0
  Constant1 : Constant  Value=Dp0
  Constant2 : Constant  Value=Kj
  Constant3 : Constant  Value=Kd
  Delay : Delay  DelayLength=1  SampleTime=Ts
  Delay1 : Delay  DelayLength=1  SampleTime=Ts
  Demux : Demux  Outputs=2
  Discrete-Time Integrator1 : DiscreteIntegrator  SampleTime=Ts  ICPrevOutput=DiscIntNeverNeededParam  ICPrevScaledInput=DiscIntNeverNeededParam
  Discrete-Time Integrator2 : DiscreteIntegrator  SampleTime=Ts  ICPrevOutput=DiscIntNeverNeededParam  ICPrevScaledInput=DiscIntNeverNeededParam
  Discrete-Time Integrator3 : DiscreteIntegrator  SampleTime=Ts  ICPrevOutput=DiscIntNeverNeededParam  ICPrevScaledInput=DiscIntNeverNeededParam
  Divide : Product  Inputs=*/
  Divide1 : Product  Inputs=*/
  Divide2 : Product  Inputs=*/
  First-Order Filter : spsFirstOrderFilterLib/First-Order Filter  FilterType=Lowpass  Tc=2*pi*Ts*10  Ts=Ts  Initialize=on  Vac_Init=[0, 0, Fg]  Vdc_Init=J0  PlotResponse=off  FreqRange="[0,  200,  1]"
  First-Order Filter1 : spsFirstOrderFilterLib/First-Order Filter  FilterType=Lowpass  Tc=2*pi*Ts*10  Ts=Ts  Initialize=on  Vac_Init=[0, 0, Fg]  Vdc_Init=Dp0  PlotResponse=off  FreqRange="[0,  200,  1]"
  Gain : Gain  Gain=1/2/pi
  Gain1 : Gain  Gain=2*pi
  Gain3 : Gain  Gain=Fnom
  Lvirtual : Gain  Gain=Lf/Zn
  MATLAB Function : MATLAB Function  TreatAsAtomicUnit=on
  PQ->pu1 : Gain  Gain=1/Pnom  SaturateOnIntegerOverflow=on  OutDataTypeStr=Inherit: Same as input  ParamDataTypeStr=Inherit: Same as input
  PQ->pu2 : Gain  Gain=1/Pnom  SaturateOnIntegerOverflow=on  OutDataTypeStr=Inherit: Same as input  ParamDataTypeStr=Inherit: Same as input
  Product{,1..6} (7 alike) : Product
  Rvirtual : Constant  Value=Rf/Zn
  Scope2 : Scope
  Selector8 : Selector  InputPortWidth=2  IndexOptions=Index vector (dialog)  Indices=[2]  OutputSizes=1
  Sum : Sum  Inputs=|+-
  Sum1 : Sum  Inputs=|++
  Sum2 : Sum  Inputs=-+-
  Sum3 : Sum  Inputs=|++
  Sum4 : Sum  Inputs=-+|
  Sum5 : Sum  Inputs=-++
  Sum6 : Sum  Inputs=|-+
  Sum7 : Sum  Inputs=|+-
  Sum8 : Sum  Inputs=|+-
  mw : Gain  Gain=100/Frequency_Droop
  nu : Gain  Gain=100/Voltage_Droop
  to-pu : Gain  Gain=1/Fnom
  to-pu1 : Gain  Gain=1/Vnom
  w0 : Constant  Value=2*pi
  Fout : Outport
  theta_out : Outport  Port=2
  Vqout : Outport  Port=3
  Vdout : Outport  Port=4
  wires:
  Fref/1 -> to-pu/1
  Sum/1 -> mw/1
  mw/1 -> Sum1/1
  Sum1/1 -> Divide/1  "Pm"
  Divide/1 -> Sum2/2  "Tm"
  Divide1/1 -> Sum2/3  "Te"
  Sum2/1 -> Divide2/1
  Divide2/1 -> [dw_dt], Discrete-Time Integrator1/1  "dw/dt"
  Discrete-Time Integrator1/1 -> [dw], Sum3/1, Product/2  "w-w0"
  [Dp] -> Product/1
  Product/1 -> Sum2/1
  w0/1 -> Sum3/2
  Gain1/1 -> Sum/1
  Discrete-Time Integrator2/1 -> theta_out/1
  to-pu/1 -> Gain1/1
  Gain/1 -> Scope2/1, Fout/1
  Sum3/1 -> Lvirtual/1, Divide1/2, Divide/2, Sum/2, Gain3/1  "w"
  Gain3/1 -> Discrete-Time Integrator2/1, Gain/1
  Discrete-Time Integrator3/1 -> 1/k/1
  Sum5/1 -> Discrete-Time Integrator3/1
  to-pu1/1 -> Sum4/2
  Selector8/1 -> Sum4/1
  VdVq/1 -> Selector8/1
  Q0/1 -> PQ->pu1/1
  nu/1 -> Sum5/2
  Sum4/1 -> nu/1
  Vref/1 -> to-pu1/1
  Qmeas/1 -> Product1/2
  Pmeas/1 -> Product2/1
  Enable/1 -> Product1/1, Product2/2
  Product2/1 -> Divide1/1
  [dw] -> Delay/1
  Demux/1 -> Product5/1, Product3/2
  Demux/2 -> Product6/1, Product4/1
  Lvirtual/1 -> Product3/1, Product4/2
  Product3/1 -> Sum6/1
  1/k/1 -> Sum6/2  "E"
  Product4/1 -> Sum8/1
  Product1/1 -> Sum5/1
  [J] -> Divide2/2
  [dw_dt] -> Delay1/1
  Delay/1 -> MATLAB Function/1(dw)
  Delay1/1 -> MATLAB Function/2(dw_dt)
  Constant/1 -> MATLAB Function/3(J0)
  Constant1/1 -> MATLAB Function/4(Dp0)
  MATLAB Function/2(Dp) -> First-Order Filter1/1
  adapativeOn/1 -> MATLAB Function/7(enable)
  Constant2/1 -> MATLAB Function/5(Kj)
  Constant3/1 -> MATLAB Function/6(Kd)
  MATLAB Function/1(J) -> First-Order Filter/1
  P0/1 -> PQ->pu2/1
  PQ->pu2/1 -> Sum1/2
  PQ->pu1/1 -> Sum5/3
  First-Order Filter/1 -> [J]
  First-Order Filter1/1 -> [Dp]
  Sum7/1 -> Vqout/1
  Product5/1 -> Sum8/2
  Rvirtual/1 -> Product5/2, Product6/2
  Product6/1 -> Sum7/2
  Sum6/1 -> Sum7/1
  Sum8/1 -> Vdout/1
  IdIq/1 -> Demux/1
